simulink model "ards_model"  (R2020b)
settings: Solver=VariableStepAuto  StartTime=0.0  StopTime=480  MaxStep=0.2  RelTol=1e-3
model workspace: external: MAT-File model_workspace.mat (data not in the file)
values from neighbouring files (symbols this model uses):
  C_a_CO2_0 = 0.54    [model_workspace.mat]
  C_a_O2_0 = 0.1974    [model_workspace.mat]
  C_v_CO2_0 = 0.72    [model_workspace.mat]
  C_v_O2_0 = 0.13    [model_workspace.mat]
  moving_average_period = 5    [model_workspace.mat]
  P_ap_0 = 15    [model_workspace.mat]
  P_as_0 = 105.55    [model_workspace.mat]
  P_default = [105.55 4 15 6]    [model_workspace.mat]
  P_vs_0 = 4    [model_workspace.mat]
  Q_0 = 4.8    [model_workspace.mat]
undefined symbols (not defined in the file or in its folder): cRS, Pinsp, VT
libraries: pid_lib x1
(part 1 of 3)
settings Model: OrderedModelArguments=off  Creator=RH  LastModifiedBy=fonck
settings DebuggingCC: SignalInfNanChecking=warning  AlgebraicLoopMsg=none  ArtificialAlgebraicLoopMsg=none  UnconnectedInputMsg=none  UnconnectedOutputMsg=none  UnconnectedLineMsg=none  UniqueDataStoreMsg=error  BusObjectLabelMismatch=none

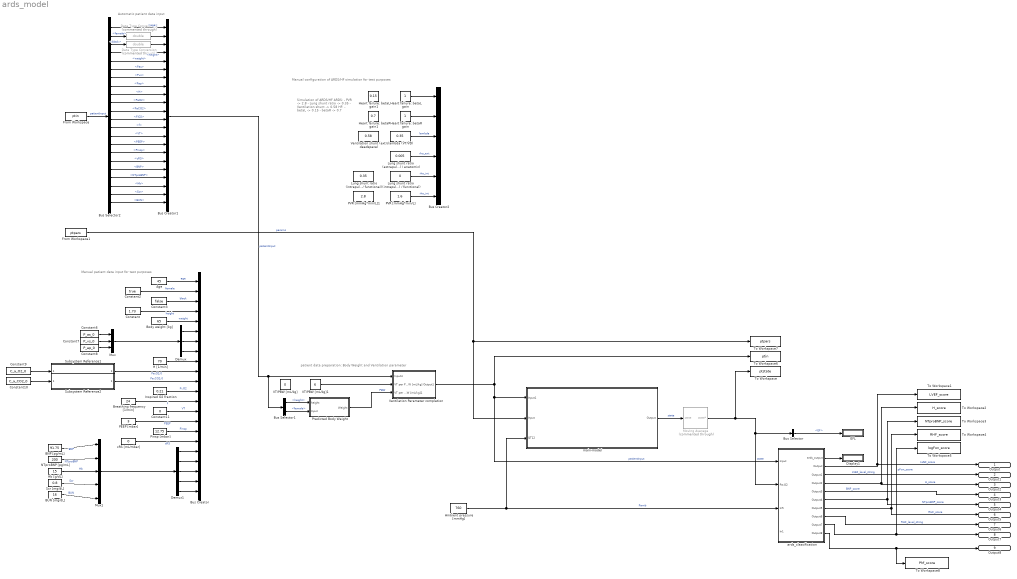
== system ards_model ==
  note: patient data preparation: Body Weight and Ventilation parameter
  note: Manual configuration of ARDS/HF simulation for test purposes
  note: Automatic patient data input
  note: Manual patient data input for test purposes
  note: Simulation of ARDS/HF
      | ARDS:
      | - PVR -> 2.8
      | - Lung shunt ratio -> 0.35
      | - Ventilation shunt -> 0.58
      | HF:
      | - betaL -> 0.15
      | - betaR -> 0.7
  Age : Constant  Value=45
  Ambient pressure [mmHg] : Constant  Value=760
  BNP [pg/mL] : Constant  Value=91.75
  BUN [mg/dL] : Constant  Value=16
  Body weight [kg] : Constant  Value=65  OutDataTypeStr=double
  Breathing frequency [1/min] : Constant  Value=24
  Bus Creator : BusCreator  Inputs=22  OutDataTypeStr=Bus: PatientInput
      settings: InheritFromInputs=off
  Bus Creator1 : BusCreator  Inputs=22  OutDataTypeStr=Bus: PatientInput
      settings: InheritFromInputs=off
  Bus Creator2 : BusCreator  Inputs=6  OutDataTypeStr=Bus: PatientParams
      settings: InheritFromInputs=off
  Bus Selector : BusSelector  OutputSignals=cvs.LV.EF
  Bus Selector1 : BusSelector  OutputSignals=height,female
  Bus Selector2 : BusSelector  OutputSignals=age,female,black,height,weight,Pas,Pvs,Pap,H,PaO2,PaCO2,FiO2,f,VT,PEEP,Pinsp,cRS,BNP,NTproBNP,Hb,Scr,BUN
  Constant : Constant  Value=1.73
  Constant10 : Constant  Value=C_a_CO2_0
  Constant11 : Constant  Value=0
  Constant2 : Constant  Value=true
  Constant3 : Constant  Value=false
  Constant6 : Constant  Value=P_as_0
  Constant7 : Constant  Value=P_vs_0
  Constant8 : Constant  Value=P_ap_0
  Constant9 : Constant  Value=C_a_O2_0
  Data Type Conversion : DataTypeConversion  Commented=through  OutDataTypeStr=double
  Data Type Conversion1 : DataTypeConversion  Commented=through  OutDataTypeStr=double
  Demux : Demux  Outputs=3
  Demux1 : Demux  Outputs=5
  Display1 : Display
  EFL : Display
  From Workspace : FromWorkspace  VariableName=ptin  OutDataTypeStr=Bus: PatientInput  OutputAfterFinalValue=Holding final value
  From Workspace1 : FromWorkspace  VariableName=ptpars  OutDataTypeStr=Bus: PatientParams  OutputAfterFinalValue=Holding final value
  H [1/min] : Constant  Value=70
  Hb [g/dL] : Constant  Value=15
  Heart failure: betaL gain : Constant
  Heart failure: betaL gain1 : Constant  Value=0.15
  Heart failure: betaR gain : Constant
  Heart failure: betaR gain1 : Constant  Value=0.7
  Inspired O2 fraction : Constant  Value=0.21
  Lung shunt ratio (extrapulmonal / anatomic) : Constant  Value=0.005
  Lung shunt ratio (intrapulmonal / functional) : Constant  Value=0
  Lung shunt ratio (intrapulmonal / functional)1 : Constant  Value=0.35
  Moving Average : Subsystem  Commented=through
  Mux : Mux  Inputs=3
  Mux1 : Mux  Inputs=5
  NTproBNP [pg/mL] : Constant  Value=200
  PEEP [mbar] : Constant  Value=3
  PVR [mmHg*min/L] : Constant  Value=1.6
  PVR [mmHg*min/L]1 : Constant  Value=2.8
  Pinsp [mbar] : Constant  Value=12.75
  Predicted Body Weight : Subsystem  TreatAsAtomicUnit=on
  Scr [mg/dL] : Constant  Value=0.8
  Subsystem Reference1 : Subsystem  ReferencedSubsystem=O2_dissociation_inv
  Subsystem Reference2 : Subsystem  ReferencedSubsystem=CO2_dissociation_inv
  To Workspace : ToWorkspace  VariableName=ptstate  SaveFormat=Timeseries  SampleTime=-1
  To Workspace1 : ToWorkspace  VariableName=LVEF_score  SaveFormat=Timeseries  SampleTime=-1
  To Workspace2 : ToWorkspace  VariableName=H_score  SaveFormat=Timeseries  SampleTime=-1
  To Workspace3 : ToWorkspace  VariableName=NTproBNP_score  SaveFormat=Timeseries  SampleTime=-1
  To Workspace4 : ToWorkspace  VariableName=RHF_score  SaveFormat=Timeseries  SampleTime=-1
  To Workspace5 : ToWorkspace  VariableName=logFon_score  SaveFormat=Timeseries  SampleTime=-1
  To Workspace6 : ToWorkspace  VariableName=ptin  SaveFormat=Timeseries  SampleTime=-1
  To Workspace7 : ToWorkspace  VariableName=ptpars  SaveFormat=Timeseries  SampleTime=-1
  To Workspace8 : ToWorkspace  VariableName=Phf_score  SaveFormat=Timeseries  SampleTime=-1
  VT/PBW [mL/kg] : Constant  Value=0
  VT/PBW [mL/kg]1 : Constant  Value=6
  Ventilation Parameter completion : Subsystem
  Ventilation shunt (extra deadspace) : Constant  Value=0.58
  ards_classification : Subsystem
  cRS [mL/mbar] : Constant  Value=0
  lambda (VT/VD) : Constant  Value=0.35
  main-model : Subsystem
  Output : Outport
  Output1 : Outport  Port=2
  Output2 : Outport  Port=3
  Output3 : Outport  Port=4
  Output4 : Outport  Port=5
  Output5 : Outport  Port=6
  Output6 : Outport  Port=7
  Output7 : Outport  Port=8
  Output8 : Outport  Port=9
  wires:
  Breathing frequency [1/min]/1 -> Bus Creator/13  "f"
  Ambient pressure [mmHg]/1 -> main-model/3(QT12), ards_classification/3(In5)  "Pamb"
  Inspired O2 fraction/1 -> Bus Creator/12  "Fi;O2"
  Constant2/1 -> Bus Creator/2  "female"
  Constant3/1 -> Bus Creator/3  "black"
  H [1/min]/1 -> Bus Creator/9
  Bus Selector1/1 -> Predicted Body Weight/1(height)  "<height>"
  Predicted Body Weight/1(Weight) -> Ventilation Parameter completion/3(VT per PBW [mL/kg]1)  "PBW"
  Bus Selector1/2 -> Predicted Body Weight/2(Input)  "<female>"
  VT/PBW [mL/kg]1/1 -> Ventilation Parameter completion/2(VT per PBW [mL/kg])
  Bus Creator1/1 -> Bus Selector1/1, Ventilation Parameter completion/1(Input4)  "patientInput"
  Body weight [kg]/1 -> Bus Creator/5  "weight"
  Age/1 -> Bus Creator/1  "age"
  Demux/1 -> Bus Creator/6
  Demux/2 -> Bus Creator/7
  Demux/3 -> Bus Creator/8
  Constant6/1 -> Mux/1
  Constant7/1 -> Mux/2
  Constant8/1 -> Mux/3
  Mux/1 -> Demux/1
  Subsystem Reference1/1 -> Bus Creator/10  "Pa;O2;0"
  Subsystem Reference2/1 -> Bus Creator/11  "Pa;CO2;0"
  Constant9/1 -> Subsystem Reference1/1
  Constant10/1 -> Subsystem Reference2/1
  Constant11/1 -> Bus Creator/14  "VT"
  PEEP [mbar]/1 -> Bus Creator/15  "PEEP"
  Pinsp [mbar]/1 -> Bus Creator/16  "Pinsp"
  cRS [mL/mbar]/1 -> Bus Creator/17  "cRS"
  Ventilation Parameter completion/1(Output1) -> To Workspace6/1, main-model/1(Input1), ards_classification/1(Input)  "patientInput"
  Scr [mg/dL]/1 -> Mux1/4  "Scr"
  NTproBNP [pg/mL]/1 -> Mux1/2  "NTproBNP"
  Hb [g/dL]/1 -> Mux1/3  "Hb"
  BNP [pg/mL]/1 -> Mux1/1  "BNP"
  Demux1/4 -> Bus Creator/21
  Demux1/1 -> Bus Creator/18
  Demux1/2 -> Bus Creator/19
  Demux1/3 -> Bus Creator/20
  Mux1/1 -> Demux1/1
  Bus Selector/1 -> EFL/1  "<EF>"
  Constant/1 -> Bus Creator/4  "height"
  main-model/1(Output) -> Moving Average/1(state)  "state"
  Moving Average/1(state*) -> To Workspace/1, Bus Selector/1, ards_classification/2(Pa;O2)  "state"
  Heart failure: betaR gain/1 -> Bus Creator2/2
  Heart failure: betaL gain/1 -> Bus Creator2/1
  lambda (VT/VD)/1 -> Bus Creator2/3  "lambda"
  Lung shunt ratio (extrapulmonal / anatomic)/1 -> Bus Creator2/4  "rho_ext"
  Lung shunt ratio (intrapulmonal / functional)/1 -> Bus Creator2/5  "rho_int"
  From Workspace1/1 -> To Workspace7/1, main-model/2(Input)  "params"
  PVR [mmHg*min/L]/1 -> Bus Creator2/6  "rho_int"
  BUN [mg/dL]/1 -> Mux1/5  "BUN"
  Demux1/5 -> Bus Creator/22
  ards_classification/2(Output) -> Output/1, To Workspace1/1  "LVEF_score"
  ards_classification/3(Output1) -> Output1/1  "LVEF_level_string"
  ards_classification/9(Output7) -> To Workspace5/1, Output7/1  "pFon_score"
  ards_classification/8(Output6) -> Output6/1  "RHF_level_string"
  ards_classification/7(Output5) -> Output5/1, To Workspace4/1  "RHF_score"
  ards_classification/6(Output4) -> Output4/1, To Workspace3/1  "NTproBNP_score"
  ards_classification/5(Output3) -> Output3/1  "BNP_score"
  ards_classification/4(Output2) -> Output2/1, To Workspace2/1  "H_score"
  Bus Selector2/21 -> Bus Creator1/21  "<Scr>"
  Bus Selector2/22 -> Bus Creator1/22  "<BUN>"
  Bus Selector2/19 -> Bus Creator1/19  "<NTproBNP>"
  Bus Selector2/20 -> Bus Creator1/20  "<Hb>"
  Bus Selector2/18 -> Bus Creator1/18  "<BNP>"
  Bus Selector2/16 -> Bus Creator1/16  "<Pinsp>"
  Bus Selector2/17 -> Bus Creator1/17  "<cRS>"
  Bus Selector2/15 -> Bus Creator1/15  "<PEEP>"
  Bus Selector2/14 -> Bus Creator1/14  "<VT>"
  Bus Selector2/12 -> Bus Creator1/12  "<FiO2>"
  Bus Selector2/11 -> Bus Creator1/11  "<PaCO2>"
  Bus Selector2/13 -> Bus Creator1/13  "<f>"
  Bus Selector2/9 -> Bus Creator1/9  "<H>"
  Bus Selector2/8 -> Bus Creator1/8  "<Pap>"
  Bus Selector2/10 -> Bus Creator1/10  "<PaO2>"
  Bus Selector2/7 -> Bus Creator1/7  "<Pvs>"
  Bus Selector2/6 -> Bus Creator1/6  "<Pas>"
  Bus Selector2/4 -> Bus Creator1/4  "<height>"
  Bus Selector2/5 -> Bus Creator1/5  "<weight>"
  Bus Selector2/1 -> Bus Creator1/1  "<age>"
  Bus Selector2/2 -> Data Type Conversion1/1  "<female>"
  Bus Selector2/3 -> Data Type Conversion/1  "<black>"
  Data Type Conversion/1 -> Bus Creator1/3
  Data Type Conversion1/1 -> Bus Creator1/2
  From Workspace/1 -> Bus Selector2/1  "patientInput"
  ards_classification/1(ards_output) -> Display1/1
  ards_classification/10(Output8) -> To Workspace8/1, Output8/1

== system ards_model/Moving Average ==
  state : Inport
  Bus to Vector : BusToVector
  Gain : Gain  Gain=1/moving_average_period
  Integrator : Integrator
  Subsystem : Subsystem  ReferencedSubsystem=patient_state_to_bus
  Subtract : Sum  Inputs=+-
  Transport Delay : TransportDelay  DelayTime=moving_average_period
  state* : Outport  OutDataTypeStr=Bus: PatientState
  wires:
  Integrator/1 -> Subtract/1, Transport Delay/1
  state/1 -> Bus to Vector/1
  Subtract/1 -> Gain/1
  Transport Delay/1 -> Subtract/2
  Bus to Vector/1 -> Integrator/1
  Gain/1 -> Subsystem/1
  Subsystem/1 -> state*/1

== system ards_model/Predicted Body Weight ==
  note: Predicted body weight
      | Source: Ventilation with lower tidal volumes [...], page 3
  height : Inport  Unit=m
  Input : Inport  Port=2  OutDataTypeStr=boolean
  Add4 : Sum  Inputs=+-
  Constant1 : Constant  Value=1.524
  Constant3 : Constant  Value=0
  Gain : Gain  Gain=91
  IfThenElse : Subsystem
  Max : MinMax  Function=max  Inputs=2
  Subtract1 : Sum
  female : Constant  Value=45.5
  male : Constant  Value=50
  Weight : Outport  Unit=kg
  wires:
  Max/1 -> Gain/1
  Constant1/1 -> Add4/2
  Gain/1 -> Subtract1/1
  Constant3/1 -> Max/2
  height/1 -> Add4/1  "height"
  Subtract1/1 -> Weight/1  "PBW"
  Add4/1 -> Max/1
  female/1 -> IfThenElse/2(then)
  male/1 -> IfThenElse/3(else)
  IfThenElse/1(out) -> Subtract1/2
  Input/1 -> IfThenElse/1(if)  "female"

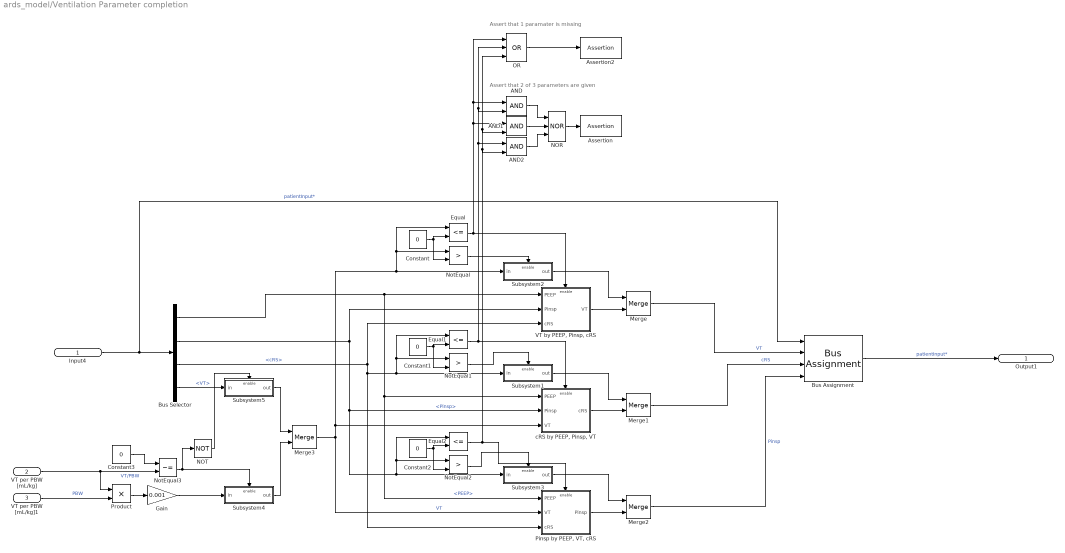
== system ards_model/Ventilation Parameter completion ==
  note: Assert that 2 of 3 parameters are given
  note: Assert that 1 paramater is missing
  Input4 : Inport  OutDataTypeStr=Bus: PatientInput
  VT per PBW [mL/kg] : Inport  Port=2  Unit=mL/kg
  VT per PBW [mL/kg]1 : Inport  Port=3  Unit=kg
  AND : Logic  IconShape=distinctive  AllPortsSameDT=off  OutDataTypeStr=boolean
  AND1 : Logic  IconShape=distinctive  AllPortsSameDT=off  OutDataTypeStr=boolean
  AND2 : Logic  IconShape=distinctive  AllPortsSameDT=off  OutDataTypeStr=boolean
  Assertion : Assertion
  Assertion2 : Assertion
  Bus Assignment : BusAssignment  AssignedSignals=VT,cRS,Pinsp
  Bus Selector : BusSelector  OutputSignals=PEEP,Pinsp,cRS,VT
  Constant{,1..3} (4 alike) : Constant  Value=0
  Equal : RelationalOperator  Operator=<=  OutDataTypeStr=boolean  RndMeth=Simplest
  Equal1 : RelationalOperator  Operator=<=  OutDataTypeStr=boolean  RndMeth=Simplest
  Equal2 : RelationalOperator  Operator=<=  OutDataTypeStr=boolean  RndMeth=Simplest
  Gain : Gain  Gain=0.001
  Merge{,1..3} (4 alike) : Merge
  NOR : Logic  Operator=NOR  Inputs=3  IconShape=distinctive  AllPortsSameDT=off  OutDataTypeStr=boolean
  NOT : Logic  Operator=NOT  IconShape=distinctive  AllPortsSameDT=off  OutDataTypeStr=boolean
  NotEqual : RelationalOperator  Operator=>  OutDataTypeStr=boolean  RndMeth=Simplest
  NotEqual1 : RelationalOperator  Operator=>  OutDataTypeStr=boolean  RndMeth=Simplest
  NotEqual2 : RelationalOperator  Operator=>  OutDataTypeStr=boolean  RndMeth=Simplest
  NotEqual3 : RelationalOperator  Operator=~=  OutDataTypeStr=boolean  RndMeth=Simplest
  OR : Logic  Operator=OR  Inputs=3  IconShape=distinctive  AllPortsSameDT=off  OutDataTypeStr=boolean
  "Pinsp by PEEP, VT, cRS" : Subsystem
  Product : Product
  Subsystem1 : Subsystem
  Subsystem2 : Subsystem
  Subsystem3 : Subsystem
  Subsystem4 : Subsystem
  Subsystem5 : Subsystem
  "VT by PEEP, Pinsp, cRS" : Subsystem
  "cRS by PEEP, Pinsp, VT" : Subsystem
  Output1 : Outport  OutDataTypeStr=Bus: PatientInput
  wires:
  Equal/1 -> OR/1, AND/1, AND1/1, "VT by PEEP, Pinsp, cRS"/Enable
  "VT by PEEP, Pinsp, cRS"/1(VT) -> Merge/2
  Bus Selector/1 -> "cRS by PEEP, Pinsp, VT"/1(PEEP), "Pinsp by PEEP, VT, cRS"/1(PEEP), "VT by PEEP, Pinsp, cRS"/1(PEEP)  "<PEEP>"
  NotEqual2/1 -> Subsystem3/Enable
  Merge3/1 -> Subsystem2/1(in), NotEqual/1, Equal/1, "cRS by PEEP, Pinsp, VT"/3(VT), "Pinsp by PEEP, VT, cRS"/2(VT)  "VT"
  Subsystem2/1(out) -> Merge/1
  Merge2/1 -> Bus Assignment/4  "Pinsp"
  Subsystem1/1(out) -> Merge1/1
  "cRS by PEEP, Pinsp, VT"/1(cRS) -> Merge1/2
  NotEqual1/1 -> Subsystem1/Enable
  "Pinsp by PEEP, VT, cRS"/1(Pinsp) -> Merge2/2
  Equal2/1 -> OR/3, AND1/2, AND2/2, "Pinsp by PEEP, VT, cRS"/Enable
  Equal1/1 -> AND2/1, OR/2, AND/2, "cRS by PEEP, Pinsp, VT"/Enable
  Merge1/1 -> Bus Assignment/3  "cRS"
  Subsystem3/1(out) -> Merge2/1
  Merge/1 -> Bus Assignment/2  "VT"
  NotEqual/1 -> Subsystem2/Enable
  AND1/1 -> NOR/2
  AND/1 -> NOR/1
  AND2/1 -> NOR/3
  NOR/1 -> Assertion/1
  OR/1 -> Assertion2/1
  Constant/1 -> Equal/2, NotEqual/2
  VT per PBW [mL/kg]/1 -> NotEqual3/2, Product/1  "VT/PBW"
  VT per PBW [mL/kg]1/1 -> Product/2  "PBW"
  Constant3/1 -> NotEqual3/1
  NotEqual3/1 -> Subsystem4/Enable, NOT/1
  Product/1 -> Gain/1
  Gain/1 -> Subsystem4/1(in)
  Subsystem5/1(out) -> Merge3/1
  Subsystem4/1(out) -> Merge3/2
  NOT/1 -> Subsystem5/Enable
  Bus Selector/4 -> Subsystem5/1(in)  "<VT>"
  Input4/1 -> Bus Assignment/1, Bus Selector/1  "patientInput*"
  Constant1/1 -> Equal1/2, NotEqual1/2
  Bus Selector/3 -> "VT by PEEP, Pinsp, cRS"/3(cRS), "Pinsp by PEEP, VT, cRS"/3(cRS), Subsystem1/1(in), NotEqual1/1, Equal1/1  "<cRS>"
  Bus Selector/2 -> "VT by PEEP, Pinsp, cRS"/2(Pinsp), Subsystem3/1(in), Equal2/1, NotEqual2/1, "cRS by PEEP, Pinsp, VT"/2(Pinsp)  "<Pinsp>"
  Constant2/1 -> NotEqual2/2, Equal2/2
  Bus Assignment/1 -> Output1/1  "patientInput*"

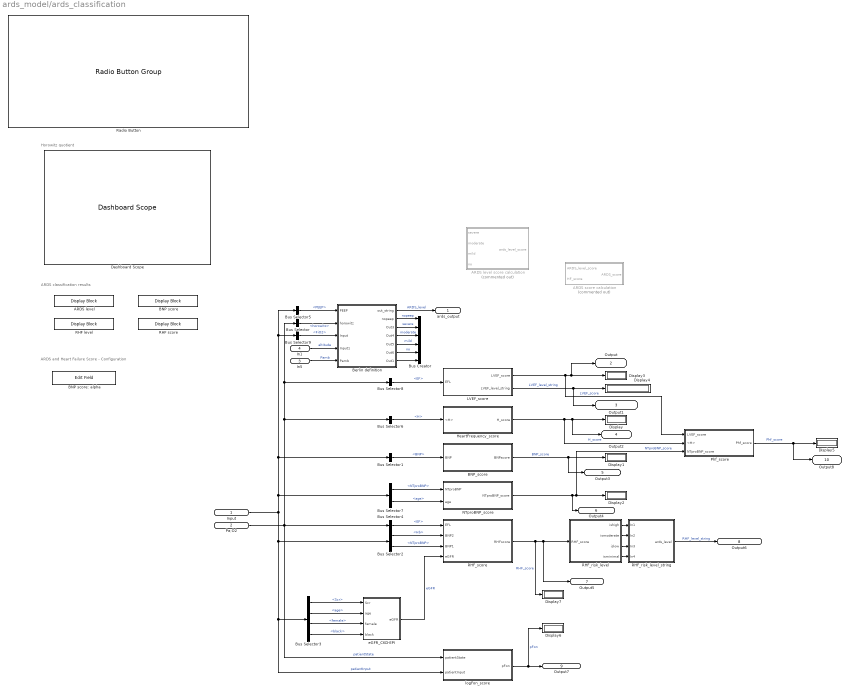
== system ards_model/ards_classification ==
  note: ARDS classification results
  note: ARDS and Heart Failure Score - Configuration
  note: Horowitz quotient
  Input : Inport  OutDataTypeStr=Bus: PatientInput
  Pa;O2 : Inport  Port=2  OutDataTypeStr=Bus: PatientState
  In5 : Inport  Port=3  Unit=mmHg
  In1 : Inport  Port=4  Unit=m
  ARDS level : DisplayBlock  LabelPosition=Hide  Format=short  Transparency=1
  ARDS level score calculation : Subsystem  Commented=on
  ARDS score calculation : Subsystem  Commented=on
  BNP score : DisplayBlock  LabelPosition=Hide  Format=short  Transparency=1
  BNP score: alpha : EditField  LabelPosition=Hide  ShowInitialText=on  Alignment=Center
  BNP_score : Subsystem
  Berlin definition : Subsystem
  Bus Creator : BusCreator  Inputs=6
  Bus Selector : BusSelector  OutputSignals=rs.horowitz
  Bus Selector1 : BusSelector  OutputSignals=BNP
  Bus Selector2 : BusSelector  OutputSignals=Hb,NTproBNP
  Bus Selector3 : BusSelector  OutputSignals=Scr,age,female,black
  Bus Selector4 : BusSelector  OutputSignals=cvs.LV.EF
  Bus Selector5 : BusSelector  OutputSignals=PEEP
  Bus Selector6 : BusSelector  OutputSignals=cvs.H
  Bus Selector7 : BusSelector  OutputSignals=NTproBNP,age
  Bus Selector8 : BusSelector  OutputSignals=cvs.LV.EF
  Bus Selector9 : BusSelector  OutputSignals=FiO2
  Dashboard Scope : DashboardScope  ShowInitialText=off  Ymin=0  Ymax=750
  Display{,1..7} (8 alike) : Display
  HeartFrequency_score : Subsystem
  LVEF_score : Subsystem
  NTproBNP_score : Subsystem
  Phf_score : Subsystem
  RHF level : DisplayBlock  LabelPosition=Hide  Format=short  Transparency=1
  RHF score : DisplayBlock  LabelPosition=Hide  Format=short  Transparency=1
  RHF_risk_level : Subsystem
  RHF_risk_level_string : Subsystem
  RHF_score : Subsystem
  Radio Button : RadioButtonGroup  LabelPosition=Hide  SelectedLabel=Pérez-Padilla et al. (altitude)  ButtonGroupName=Horowitz correction mode
      settings: Values={{'Pérez-Padilla et al. (altitude)', 'Pérez-Padilla et al. (Pamb)', 'Berlin Definition (original)', 'Berlin Definition (reciprocal)'}, [1 2 3 4]}
  eGFR_CKD-EPI : Subsystem
  logFon_score : Subsystem
  ards_output : Outport
  Output : Outport  Port=2
  Output1 : Outport  Port=3
  Output2 : Outport  Port=4
  Output3 : Outport  Port=5
  Output4 : Outport  Port=6
  Output5 : Outport  Port=7
  Output6 : Outport  Port=8
  Output7 : Outport  Port=9
  Output8 : Outport  Port=10
  wires:
  Bus Selector1/1 -> BNP_score/1(BNP)  "<BNP>"
  Berlin definition/1(out_string) -> ards_output/1  "ARDS_level"
  Pa;O2/1 -> logFon_score/1(patientState), Bus Selector8/1, Bus Selector/1, Bus Selector6/1, Bus Selector4/1  "patientState"
  In5/1 -> Berlin definition/5(Pamb)  "Pamb"
  Bus Selector/1 -> Berlin definition/2(horowitz)  "<horowitz>"
  RHF_risk_level/1(ishigh) -> RHF_risk_level_string/1(In1)
  RHF_risk_level/2(ismoderate) -> RHF_risk_level_string/2(In2)
  RHF_risk_level/3(islow) -> RHF_risk_level_string/3(In3)
  RHF_risk_level/4(isminimal) -> RHF_risk_level_string/4(In4)
  Bus Selector2/1 -> RHF_score/2(BNP2)  "<Hb>"
  Bus Selector2/2 -> RHF_score/3(BNP1)  "<NTproBNP>"
  eGFR_CKD-EPI/1(eGFR) -> RHF_score/4(eGFR)  "eGFR"
  RHF_score/1(RHFscore) -> Display7/1, Output5/1, RHF_risk_level/1(RHF_score)  "RHF_score"
  Input/1 -> Bus Selector1/1, Bus Selector9/1, Bus Selector5/1, Bus Selector7/1, Bus Selector2/1, logFon_score/2(patientInput), Bus Selector3/1  "patientInput"
  Bus Selector3/1 -> eGFR_CKD-EPI/1(Scr)  "<Scr>"
  Bus Selector3/2 -> eGFR_CKD-EPI/2(age)  "<age>"
  Bus Selector3/4 -> eGFR_CKD-EPI/4(black)  "<black>"
  Bus Selector3/3 -> eGFR_CKD-EPI/3(female)  "<female>"
  Berlin definition/2(nopeep) -> Bus Creator/1  "nopeep"
  Berlin definition/3(Out3) -> Bus Creator/2  "severe"
  Berlin definition/4(Out4) -> Bus Creator/3  "moderate"
  Berlin definition/5(Out5) -> Bus Creator/4  "mild"
  Berlin definition/6(Out6) -> Bus Creator/5  "no"
  Berlin definition/7(Out1) -> Bus Creator/6
  Bus Selector4/1 -> RHF_score/1(EFL)  "<EF>"
  Bus Selector5/1 -> Berlin definition/1(PEEP)  "<PEEP>"
  Bus Selector6/1 -> HeartFrequency_score/1(<H>)  "<H>"
  Bus Selector7/1 -> NTproBNP_score/1(NTproBNP)  "<NTproBNP>"
  Bus Selector7/2 -> NTproBNP_score/2(age)  "<age>"
  HeartFrequency_score/1(H_score) -> Phf_score/2(<H>), Output2/1, Display/1  "H_score"
  BNP_score/1(BNPscore) -> Output3/1, Display1/1  "BNP_score"
  NTproBNP_score/1(NTproBNP_score) -> Phf_score/3(NTproBNP_score), Display2/1, Output4/1  "NTproBNP_score"
  LVEF_score/1(LVEF_score) -> Display3/1, Output/1, Phf_score/1(LVEF_score)  "LVEF_score"
  LVEF_score/2(LVEF_level_string) -> Output1/1, Display4/1  "LVEF_level_string"
  Bus Selector8/1 -> LVEF_score/1(EFL)  "<EF>"
  RHF_risk_level_string/1(ards_level) -> Output6/1  "RHF_level_string"
  logFon_score/1(pFon) -> Display6/1, Output7/1  "pFon"
  Bus Selector9/1 -> Berlin definition/3(Input)  "<FiO2>"
  In1/1 -> Berlin definition/4(Input1)  "altitude"
  Phf_score/1(Phf_score) -> Output8/1, Display5/1  "Phf_score"

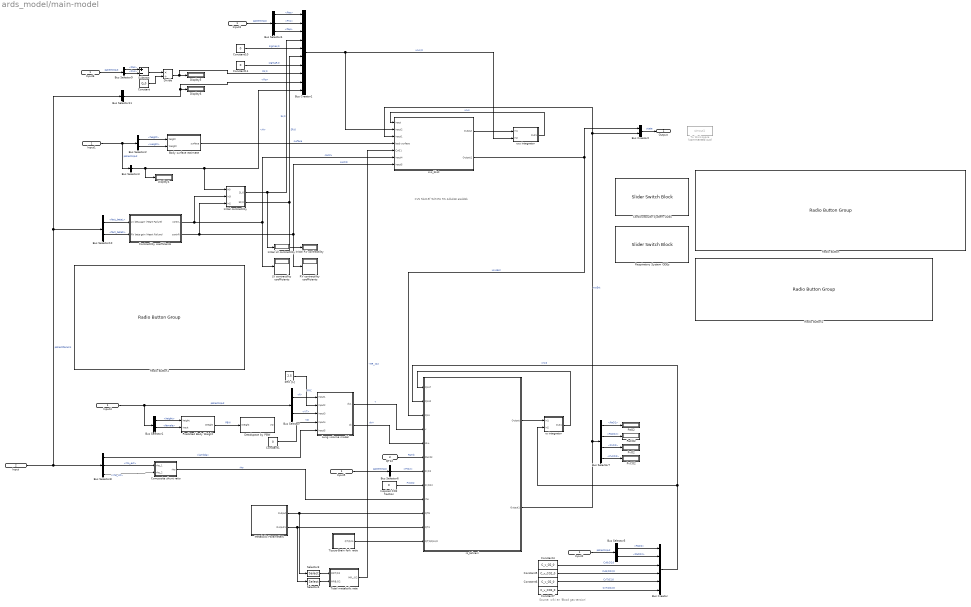
== system ards_model/main-model ==
  note: Source: wiki en 'Blood gas tension'
  note: CVS 5b215f 9d729c
      | RS 4dbd38 a6dd8b
  Input1 : Inport  OutDataTypeStr=Bus: PatientInput
  Input : Inport  Port=2  OutDataTypeStr=Bus: PatientParams  PortDimensions=6
  QT12 : Inport  Port=3  Unit=mmHg
  Body surface estimate : Subsystem  TreatAsAtomicUnit=on
  Bus Creator : BusCreator  Inputs=6  OutDataTypeStr=Bus: RespiratoryState
      settings: InheritFromInputs=off
  Bus Creator1 : BusCreator  Inputs=10  OutDataTypeStr=Bus: CardioVascularState
      settings: InheritFromInputs=off
  Bus Creator2 : BusCreator  Inputs=2  OutDataTypeStr=Bus: PatientState
      settings: InheritFromInputs=off
  Bus Selector : BusSelector  OutputSignals=f,VT
  Bus Selector1 : BusSelector  OutputSignals=height,female
  Bus Selector10 : BusSelector  OutputSignals=fact_betaL,fact_betaR
  Bus Selector11 : BusSelector  OutputSignals=Rp
  Bus Selector2 : BusSelector  OutputSignals=height,weight
  Bus Selector3 : BusSelector  OutputSignals=H
  Bus Selector4 : BusSelector  OutputSignals=Pas,Pvs,Pap
  Bus Selector5 : BusSelector  OutputSignals=PaO2,PaCO2
  Bus Selector6 : BusSelector  OutputSignals=FiO2
  Bus Selector7 : BusSelector  OutputSignals=PaO2,PaCO2,PvO2,PvCO2
  Bus Selector8 : BusSelector  OutputSignals=lambda,rho_ext,rho_int
  Bus Selector9 : BusSelector  OutputSignals=Pas,Pvs
  Cardiovascular System ODEs : SliderSwitchBlock
      settings: Values={{'Off', 'On'}, [0 1]}
  Composite shunt ratio : Subsystem
  Constant : Constant  Value=Q_0
  Constant1 : Constant  Value=0
  Constant10 : Constant  Value=0
  Constant11 : Constant  Value=0
  Constant4 : Constant  Value=C_v_O2_0
  Constant5 : Constant  Value=C_v_CO2_0
  Constant6 : Constant  Value=C_v_O2_0
  Constant7 : Constant  Value=C_v_CO2_0
  Contractility coefficients : Subsystem
  Deadspace by PBW : Subsystem  TreatAsAtomicUnit=on
  Display4 : Display
  Display5 : Display
  Display6 : Display
  Divide : Product  Inputs=*/
  FRC [L] : Constant  Value=2.5
  Initial LV contractility : Display
  Initial RV contractility : Display
  Initial contractility : Subsystem
  Input{2..6} (5 alike) : InportShadow  OutDataTypeStr=Bus: PatientInput
  Inspired CO2 fraction : Constant  Value=0
  LV contractility coefficients : Display
  Lung volume model : Subsystem  TreatAsAtomicUnit=on
  Metabolic Parameters : Subsystem
  PaCO2 : Display
  PaO2 : Display
  Predicted Body Weight : Subsystem  TreatAsAtomicUnit=on
  PvCO2 : Display
  PvO2 : Display
  RV contractility coefficients : Display
  Radio Button : RadioButtonGroup  LabelPosition=Hide  SelectedLabel=ODE from [BKST (1.27)]: By Metabolic rates and Ca;O2  ButtonGroupName=Systemic vascular resistance: Calculation mode
      settings: Values={{'Constant', 'Linear relation from [BKST (1.24)]: By Cv;O2', 'ODE from [BKST (1.27)]: By Metabolic rates and Ca;O2'}, [0 1 2]}
  Radio Button1 : RadioButtonGroup  LabelPosition=Hide  SelectedLabel=from table 3.1 (healthy)  ButtonGroupName=Contractility coefficient selection (see [BKST] table 1.5)
      settings: Values={{'without QL measurements', 'with QL measurements', 'with QL measurements, "exact" gradients', 'from table 3.1 (healthy)', 'from table 3.1 (Heart Failure)'}, [1 2 3 4 5]}
  Radio Button2 : RadioButtonGroup  LabelPosition=Hide  SelectedLabel=Linear relationship with Heart Frequency (H)  ButtonGroupName=Heart Contractility: Calculation mode
      settings: Values={{'Linear relationship with Heart Frequency (H)', 'Second-order ODE'}, [0 1]}
  Respiratory System ODEs : SliderSwitchBlock
      settings: Values={{'Off', 'On'}, [0 1]}
  Selector3 : Selector  InputPortWidth=3  IndexOptions=Index vector (dialog)  Indices=2  OutputSizes=1
  Selector4 : Selector  InputPortWidth=3  IndexOptions=Index vector (dialog)  Indices=2  OutputSizes=1
  Subtract : Sum  Inputs=+-
  Tissue-Brain fork ratio : Subsystem
  To Workspace : ToWorkspace  Commented=on  VariableName=simout1  SaveFormat=Timeseries  SampleTime=-1
      settings: MaxDataPoints=1
  Total metabolic rate : Subsystem
  cvs integrator : Subsystem
  cvs_bkst : Subsystem
  rs integrator : Subsystem
  rs_tehrani : Subsystem  TreatAsAtomicUnit=on
  Output : Outport  OutDataTypeStr=Bus: PatientState
  wires:
  Divide/1 -> Bus Creator1/8, Display5/1  "Rs;0"
  Bus Selector9/2 -> Subtract/2  "<Pvs>"
  Bus Selector9/1 -> Subtract/1  "<Pas>"
  Input5/1 -> Bus Selector6/1  "patientInput"
  Input2/1 -> Bus Selector5/1  "patientInput"
  Bus Selector/2 -> Lung volume model/3(Input3)  "<VT>"
  Bus Selector7/1 -> PaO2/1  "<PaO2>"
  Bus Selector7/3 -> PvO2/1  "<PvO2>"
  Input1/1 -> Bus Selector2/1, Bus Selector3/1  "patientInput"
  Bus Selector7/2 -> PaCO2/1  "<PaCO2>"
  Bus Selector5/2 -> Bus Creator/2  "<PaCO2>"
  cvs_bkst/2(Output1) -> Bus Creator2/1, rs_tehrani/3(Qco)  "xcvsExt"
  Bus Creator2/1 -> Output/1  "state"
  Contractility coefficients/1(contrL) -> cvs_bkst/6(Input4), LV contractility coefficients/1, Initial contractility/2(In3)  "contrL"
  cvs integrator/1(Out1) -> cvs_bkst/1(Input)  "xcvs"
  Contractility coefficients/2(contrR) -> cvs_bkst/7(Input5), RV contractility coefficients/1, Initial contractility/3(In2)  "contrR"
  cvs_bkst/1(Output) -> cvs integrator/1(In1)
  rs_tehrani/2(Output1) -> Bus Creator2/2, cvs_bkst/3(Input1), Bus Selector7/1  "xrsExt"
  Bus Selector4/3 -> Bus Creator1/3  "<Pap>"
  Bus Selector4/1 -> Bus Creator1/1  "<Pas>"
  Bus Selector11/1 -> Bus Creator1/9, Display6/1  "<Rp>"
  Bus Creator1/1 -> cvs integrator/2(In2), cvs_bkst/2(Input2)  "xcvs;0"
  Total metabolic rate/1(MR_;O2) -> cvs_bkst/5(CvO1)  "-MR_;O2"
  Bus Selector7/4 -> PvCO2/1  "<PvCO2>"
  Constant10/1 -> Bus Creator1/5  "sigmaL;0"
  Bus Selector10/1 -> Contractility coefficients/1(LV beta gain (Heart Failure))  "<fact_betaL>"
  Bus Selector1/2 -> Predicted Body Weight/2(Input)  "<female>"
  Constant11/1 -> Bus Creator1/7  "sigmaR;0"
  Bus Selector4/2 -> Bus Creator1/2  "<Pvs>"
  Initial contractility/1(SL;0) -> Initial LV contractility/1, Bus Creator1/4  "SL;0"
  Bus Selector10/2 -> Contractility coefficients/2(RV beta gain (Heart Failure))  "<fact_betaR>"
  Input3/1 -> Bus Selector4/1  "patientInput"
  Input6/1 -> Bus Selector9/1  "patientInput"
  rs integrator/1(Out1) -> rs_tehrani/1(Qco7)
  Bus Selector5/1 -> Bus Creator/1  "<PaO2>"
  rs_tehrani/1(Output) -> rs integrator/1(In1)
  Bus Selector1/1 -> Predicted Body Weight/1(height)  "<height>"
  Constant7/1 -> Bus Creator/6  "CvT;CO2;0"
  Constant/1 -> Divide/2
  Bus Selector/1 -> Lung volume model/1(Input1)  "<f>"
  FRC [L]/1 -> Lung volume model/2(Input2)  "FRC"
  Lung volume model/1(dv1) -> rs_tehrani/4(v)  "v"
  Constant1/1 -> Lung volume model/4(Input4)  "VD"
  Bus Selector2/1 -> Body surface estimate/1(height)  "<height>"
  Subtract/1 -> Divide/1
  Lung volume model/2(dv) -> rs_tehrani/5(dv+)  "dv+"
  QT12/1 -> rs_tehrani/6(Pamb*)  "Pamb"
  Constant5/1 -> Bus Creator/4  "CvB;CO2;0"
  Predicted Body Weight/1(Weight) -> Deadspace by PBW/1(Weight)  "PBW"
  Bus Selector8/1 -> Lung volume model/5(Input5)  "<lambda>"
  Constant4/1 -> Bus Creator/3  "CvB;O2;0"
  Body surface estimate/1(surface) -> cvs_bkst/4(body surface)  "surface"
  Bus Selector3/1 -> Display4/1, Bus Creator1/10, Initial contractility/1(H0)  "<H>"
  Initial contractility/2(SR;0) -> Initial RV contractility/1, Bus Creator1/6  "SR;0"
  Bus Selector2/2 -> Body surface estimate/2(Weight)  "<weight>"
  Input/1 -> Bus Selector11/1, Bus Selector10/1, Bus Selector8/1  "patientParams"
  Tissue-Brain fork ratio/1(QT/Qco) -> rs_tehrani/12(QT;0/Qco;0)
  Bus Creator/1 -> rs integrator/2(In2), rs_tehrani/2(Qco2)  "xrs;0"
  Bus Selector8/3 -> Composite shunt ratio/2(rho_2)  "<rho_int>"
  Input4/1 -> Bus Selector1/1, Bus Selector/1  "patientInput"
  Constant6/1 -> Bus Creator/5  "CvT;O2;0"
  Composite shunt ratio/1(rho) -> rs_tehrani/9(rho)  "rho"
  Bus Selector8/2 -> Composite shunt ratio/1(rho_1)  "<rho_ext>"
  Bus Selector6/1 -> rs_tehrani/7(Fi;O2)  "<FiO2>"
  Inspired CO2 fraction/1 -> rs_tehrani/8(Fi;CO2)  "Fi;CO2"
  Selector3/1 -> Total metabolic rate/1(MRT;O2)
  Selector4/1 -> Total metabolic rate/2(MRB;O2)
  Metabolic Parameters/1(Output) -> Selector3/1, rs_tehrani/10(QT8)
  Metabolic Parameters/2(Output1) -> Selector4/1, rs_tehrani/11(QT4)

== system ards_model/Predicted Body Weight/IfThenElse ==
  if : Inport  OutDataTypeStr=boolean
  then : Inport  Port=2
  else : Inport  Port=3
  Merge : Merge
  NOT : Logic  Operator=NOT  IconShape=distinctive  AllPortsSameDT=off  OutDataTypeStr=boolean
  Subsystem1 : Subsystem
  Subsystem2 : Subsystem
  out : Outport
  wires:
  then/1 -> Subsystem1/1(in)
  Subsystem2/1(out) -> Merge/2
  if/1 -> NOT/1, Subsystem1/Enable
  else/1 -> Subsystem2/1(in)
  Subsystem1/1(out) -> Merge/1
  NOT/1 -> Subsystem2/Enable
  Merge/1 -> out/1

== system ards_model/Ventilation Parameter completion/Pinsp by PEEP, VT, cRS ==
  PEEP : Inport  Unit=mbar
  VT : Inport  Port=2  Unit=L
  cRS : Inport  Port=3  Unit=mL/mbar
  Enable : EnablePort
  Add : Sum
  Divide1 : Product  Inputs=*/
  Gain : Gain  Gain=0.001
  Pinsp : Outport  Unit=mbar
  wires:
  Divide1/1 -> Add/2
  cRS/1 -> Gain/1
  PEEP/1 -> Add/1
  Add/1 -> Pinsp/1  "Pinsp"
  VT/1 -> Divide1/1
  Gain/1 -> Divide1/2

== system ards_model/Ventilation Parameter completion/Subsystem1 ==
  in : Inport
  Enable : EnablePort
  out : Outport
  wires:
  in/1 -> out/1

== system ards_model/Ventilation Parameter completion/Subsystem2 ==
  in : Inport
  Enable : EnablePort
  out : Outport
  wires:
  in/1 -> out/1

== system ards_model/Ventilation Parameter completion/Subsystem3 ==
  in : Inport
  Enable : EnablePort
  out : Outport
  wires:
  in/1 -> out/1

== system ards_model/Ventilation Parameter completion/Subsystem4 ==
  in : Inport
  Enable : EnablePort
  out : Outport
  wires:
  in/1 -> out/1

== system ards_model/Ventilation Parameter completion/Subsystem5 ==
  in : Inport
  Enable : EnablePort
  out : Outport
  wires:
  in/1 -> out/1

== system ards_model/Ventilation Parameter completion/VT by PEEP, Pinsp, cRS ==
  PEEP : Inport  Unit=mbar
  Pinsp : Inport  Port=2  Unit=mbar
  cRS : Inport  Port=3  Unit=mL/mbar
  Enable : EnablePort
  Gain : Gain  Gain=0.001
  Product : Product
  Subtract : Sum  Inputs=-+
  VT : Outport  Unit=L
  wires:
  Product/1 -> VT/1  "VT"
  Subtract/1 -> Product/1
  Pinsp/1 -> Subtract/2
  PEEP/1 -> Subtract/1
  cRS/1 -> Gain/1
  Gain/1 -> Product/2

== system ards_model/Ventilation Parameter completion/cRS by PEEP, Pinsp, VT ==
  PEEP : Inport  Unit=mbar
  Pinsp : Inport  Port=2  Unit=mbar
  VT : Inport  Port=3  Unit=L
  Enable : EnablePort
  Divide : Product  Inputs=*/
  Gain : Gain  Gain=1000
  Subtract1 : Sum  Inputs=+-
  cRS : Outport  Unit=mL/mbar
  wires:
  VT/1 -> Divide/1
  Subtract1/1 -> Divide/2
  Pinsp/1 -> Subtract1/1
  PEEP/1 -> Subtract1/2
  Divide/1 -> Gain/1  "cRS"
  Gain/1 -> cRS/1

== system ards_model/ards_classification/ARDS level score calculation ==
  severe : Inport
  moderate : Inport  Port=2
  mild : Inport  Port=3
  no : Inport  Port=4
  ARDS level score: mild ARDS : EditField  LabelPosition=Hide  ShowInitialText=on  Alignment=Center
  ARDS level score: moderate ARDS : EditField  LabelPosition=Hide  ShowInitialText=on  Alignment=Center
  ARDS level score: no ARDS : EditField  LabelPosition=Hide  ShowInitialText=on  Alignment=Center
  ARDS level score: severe ARDS : EditField  LabelPosition=Hide  ShowInitialText=on  Alignment=Center
  ARDS score: alpha : EditField  LabelPosition=Hide  ShowInitialText=on  Alignment=Center
  Add : Sum
  Constant : Constant
  Constant1 : Constant
  Constant2 : Constant  Value=0.9
  Constant3 : Constant  Value=0.7
  Constant4 : Constant  Value=0
  Gain : Gain  Gain=2
  Merge : Merge  Inputs=4
  Product : Product
  Subsystem : Subsystem
  Subsystem1 : Subsystem
  Subsystem2 : Subsystem
  Subsystem3 : Subsystem
  Subtract : Sum  Inputs=+-
  alpha : Constant  Value=0.05
  ards_level_score : Outport  Unit=1
  wires:
  severe/1 -> Subsystem/Enable
  Subsystem/1(out) -> Merge/1
  Constant3/1 -> Subsystem2/1(in)
  Subsystem3/1(out) -> Merge/4
  Subsystem2/1(out) -> Merge/3
  Subsystem1/1(out) -> Merge/2
  Constant1/1 -> Subtract/1
  mild/1 -> Subsystem2/Enable
  alpha/1 -> Gain/1, Add/1
  Constant2/1 -> Subsystem1/1(in)
  no/1 -> Subsystem3/Enable
  moderate/1 -> Subsystem1/Enable
  Add/1 -> ards_level_score/1  "ARDS_level_score"
  Constant/1 -> Subsystem/1(in)
  Constant4/1 -> Subsystem3/1(in)
  Merge/1 -> Product/2
  Product/1 -> Add/2
  Subtract/1 -> Product/1
  Gain/1 -> Subtract/2

== system ards_model/ards_classification/ARDS score calculation ==
  ARDS_level_score : Inport  Unit=1
  HF_score : Inport  Port=2  Unit=1
  ARDS score: HF score gain : EditField  LabelPosition=Hide  ShowInitialText=on  Alignment=Center
  Constant : Constant
  Gain : Gain  Gain=0.75
  Product : Product
  Subtract : Sum  Inputs=+-
  ARDS_score : Outport  Unit=1
  wires:
  HF_score/1 -> Gain/1
  Constant/1 -> Subtract/1
  Subtract/1 -> Product/2  "no_HF_score"
  ARDS_level_score/1 -> Product/1
  Gain/1 -> Subtract/2
  Product/1 -> ARDS_score/1  "ARDS_score"

== system ards_model/ards_classification/BNP_score ==
  note: BNP Score
      | depending on the BNP input value, this subsystem calculates a score between 0 and 1.
      | 0 means no heart failure, 1 means heart failure.
      | The parameter lambda sets a minimum error, limiting the result to the interval [lambda, 1-lambda].
      | BNP values below the rule-out bound (35 pg/mL) yield a minimum score (lambda).
      | BNP values above the rule-in bound (400 pg/mL) yield a maximum score (1-lambda).
      | For values inbetween, a linear slope is generated, determined by the above boundary values.
      |
      | Source for rule-out / rule-in bounds: Zwei kardiale Marker werden "erwachsen"
  BNP : Inport  Unit=pg/mL
  BNP rule-in bound [pg/mL] : Constant  Value=400
  BNP rule-out bound [pg/mL] : Constant  Value=35
  BNP score: alpha : Constant  Value=0.05
  Constant : Constant
  Subsystem2 : Subsystem  ReferencedSubsystem=linear_slope_score
  Subtract : Sum  Inputs=+-
  BNPscore : Outport  Unit=1
  wires:
  BNP rule-out bound [pg/mL]/1 -> Subsystem2/2  "bound_ruleOut"
  Subtract/1 -> Subsystem2/5  "beta"
  BNP/1 -> Subsystem2/1
  BNP rule-in bound [pg/mL]/1 -> Subsystem2/3  "bound_ruleIn"
  Constant/1 -> Subtract/1
  Subsystem2/1 -> BNPscore/1
  BNP score: alpha/1 -> Subsystem2/4, Subtract/2  "alpha"

== system ards_model/ards_classification/Berlin definition ==
  PEEP : Inport  Unit=mbar
  horowitz : Inport  Port=2  Unit=mmHg
  Input : Inport  Port=3  Unit=1
  Input1 : Inport  Port=4  Unit=m
  Pamb : Inport  Port=5  Unit=mmHg
  Display : Display
  NOT : Logic  Operator=NOT  IconShape=distinctive  AllPortsSameDT=off  OutDataTypeStr=boolean
  PEEP bound : Subsystem
  ards_level : Subsystem
  out_string : Outport
  nopeep : Outport  Port=2
  Out3 : Outport  Port=3
  Out4 : Outport  Port=4
  Out5 : Outport  Port=5
  Out6 : Outport  Port=6
  Out1 : Outport  Port=7
  wires:
  Pamb/1 -> ards_level/4(Pamb)  "Pamb"
  ards_level/3(no) -> Out6/1  "no"
  NOT/1 -> nopeep/1  "nopeep"
  horowitz/1 -> ards_level/1(horowitz)  "horowitz"
  PEEP/1 -> PEEP bound/1(PEEP)  "PEEP"
  ards_level/4(mild) -> Out5/1  "mild"
  ards_level/5(moderate) -> Out4/1  "moderate"
  PEEP bound/1(Out1) -> ards_level/5(Input), Display/1, NOT/1  "ispeep"
  ards_level/6(severe) -> Out3/1  "severe"
  ards_level/1(Out1) -> out_string/1  "ARDS_level"
  ards_level/2(ards) -> Out1/1  "ards"
  Input/1 -> ards_level/2(Fi;O2)  "Fi;O2"
  Input1/1 -> ards_level/3(altitude)  "altitude"

== system ards_model/ards_classification/HeartFrequency_score ==
  <H> : Inport
  Constant : Constant  Value=75
  Constant1 : Constant  Value=200
  Constant2 : Constant  Value=0.2
  Constant3 : Constant  Value=0.5
  Subsystem2 : Subsystem  ReferencedSubsystem=linear_slope_score
  H_score : Outport
  wires:
  Subsystem2/1 -> H_score/1  "H_score"
  Constant1/1 -> Subsystem2/3
  Constant3/1 -> Subsystem2/5
  Constant/1 -> Subsystem2/2
  Constant2/1 -> Subsystem2/4
  <H>/1 -> Subsystem2/1  "H"

== system ards_model/ards_classification/LVEF_score ==
  EFL : Inport  Unit=1
  Constant1 : Constant  Value=0.5
  Constant2 : Constant  Value=0.3
  Constant7 : Constant  Value=0.4
  Constant8 : Constant  Value=0.5
  Enabled Subsystem : Subsystem  TreatAsAtomicUnit=on
  Enabled Subsystem1 : Subsystem  TreatAsAtomicUnit=on
  Enabled Subsystem2 : Subsystem  TreatAsAtomicUnit=on
  GreaterThan : RelationalOperator  Operator=>  OutDataTypeStr=boolean  RndMeth=Simplest
  LVEF score: max score (at EF < 30%) : Constant  Value=0.95
  LVEF score: min score (at EF > 50%) : Constant  Value=0.05
  Less Than : RelationalOperator  Operator=<  OutDataTypeStr=boolean  RndMeth=Simplest
  Merge : Merge  Inputs=3
  NOR : Logic  Operator=NOR  IconShape=distinctive  AllPortsSameDT=off  OutDataTypeStr=boolean
  String Constant : StringConstant  String="\"reduced LVEF\""
  String Constant1 : StringConstant  String="\"moderate LVEF\""
  String Constant2 : StringConstant  String="\"preserved LVEF\""
  Subsystem2 : Subsystem  ReferencedSubsystem=linear_slope_score
  LVEF_score : Outport  Unit=1
  LVEF_level_string : Outport  Port=2  Unit=1
  wires:
  LVEF score: max score (at EF < 30%)/1 -> Subsystem2/4  "alpha"
  Subsystem2/1 -> LVEF_score/1
  EFL/1 -> Subsystem2/1, GreaterThan/1, Less Than/1
  Enabled Subsystem/1(Out1) -> Merge/1
  Enabled Subsystem1/1(Out1) -> Merge/2
  Enabled Subsystem2/1(Out1) -> Merge/3
  Merge/1 -> LVEF_level_string/1
  GreaterThan/1 -> Enabled Subsystem2/Enable, NOR/2
  Constant8/1 -> GreaterThan/2
  Constant7/1 -> Less Than/2
  Less Than/1 -> NOR/1, Enabled Subsystem/Enable
  String Constant/1 -> Enabled Subsystem/1(In1)
  String Constant2/1 -> Enabled Subsystem2/1(In1)
  String Constant1/1 -> Enabled Subsystem1/1(In1)
  NOR/1 -> Enabled Subsystem1/Enable
  Constant1/1 -> Subsystem2/3
  Constant2/1 -> Subsystem2/2
  LVEF score: min score (at EF > 50%)/1 -> Subsystem2/5  "beta"

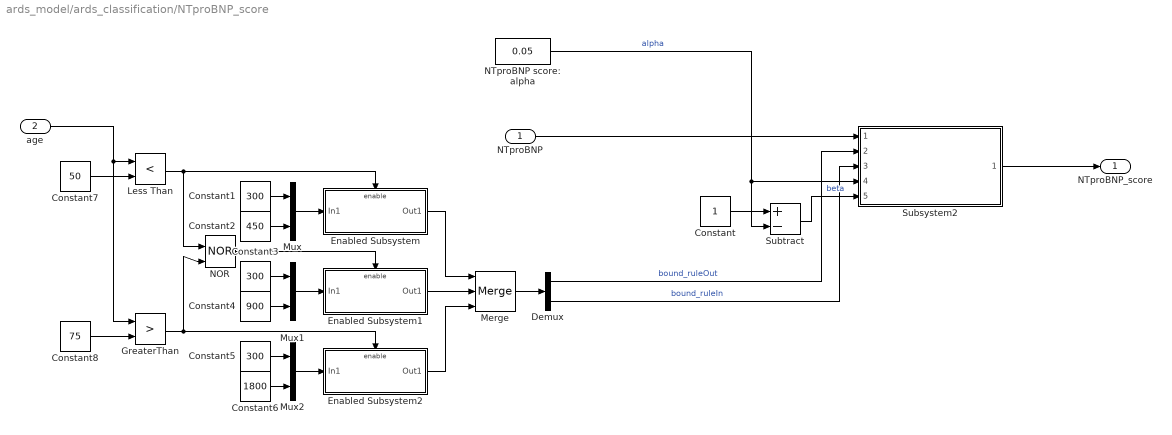
== system ards_model/ards_classification/NTproBNP_score ==
  NTproBNP : Inport  Unit=pg/mL
  age : Inport  Port=2
  Constant : Constant
  Constant1 : Constant  Value=300
  Constant2 : Constant  Value=450
  Constant3 : Constant  Value=300
  Constant4 : Constant  Value=900
  Constant5 : Constant  Value=300
  Constant6 : Constant  Value=1800
  Constant7 : Constant  Value=50
  Constant8 : Constant  Value=75
  Demux : Demux  Outputs=2
  Enabled Subsystem : Subsystem  TreatAsAtomicUnit=on
  Enabled Subsystem1 : Subsystem  TreatAsAtomicUnit=on
  Enabled Subsystem2 : Subsystem  TreatAsAtomicUnit=on
  GreaterThan : RelationalOperator  Operator=>  OutDataTypeStr=boolean  RndMeth=Simplest
  Less Than : RelationalOperator  Operator=<  OutDataTypeStr=boolean  RndMeth=Simplest
  Merge : Merge  Inputs=3
  Mux : Mux  Inputs=2
  Mux1 : Mux  Inputs=2
  Mux2 : Mux  Inputs=2
  NOR : Logic  Operator=NOR  IconShape=distinctive  AllPortsSameDT=off  OutDataTypeStr=boolean
  NTproBNP score: alpha : Constant  Value=0.05
  Subsystem2 : Subsystem  ReferencedSubsystem=linear_slope_score
  Subtract : Sum  Inputs=+-
  NTproBNP_score : Outport  Unit=1
  wires:
  NTproBNP score: alpha/1 -> Subtract/2, Subsystem2/4  "alpha"
  Subsystem2/1 -> NTproBNP_score/1
  Constant/1 -> Subtract/1
  Demux/2 -> Subsystem2/3  "bound_ruleIn"
  NTproBNP/1 -> Subsystem2/1
  Subtract/1 -> Subsystem2/5  "beta"
  Demux/1 -> Subsystem2/2  "bound_ruleOut"
  age/1 -> GreaterThan/1, Less Than/1
  Constant1/1 -> Mux/1
  Constant2/1 -> Mux/2
  Mux/1 -> Enabled Subsystem/1(In1)
  Enabled Subsystem/1(Out1) -> Merge/1
  Mux1/1 -> Enabled Subsystem1/1(In1)
  Constant4/1 -> Mux1/2
  Enabled Subsystem1/1(Out1) -> Merge/2
  Constant6/1 -> Mux2/2
  Mux2/1 -> Enabled Subsystem2/1(In1)
  Enabled Subsystem2/1(Out1) -> Merge/3
  Merge/1 -> Demux/1
  GreaterThan/1 -> NOR/2, Enabled Subsystem2/Enable
  Constant8/1 -> GreaterThan/2
  Constant7/1 -> Less Than/2
  Less Than/1 -> NOR/1, Enabled Subsystem/Enable
  NOR/1 -> Enabled Subsystem1/Enable
  Constant3/1 -> Mux1/1
  Constant5/1 -> Mux2/1

== system ards_model/ards_classification/Phf_score ==
  LVEF_score : Inport
  <H> : Inport  Port=2
  NTproBNP_score : Inport  Port=3
  Add : Sum  Inputs=+++
  Constant : Constant  Value=3
  Divide : Product  Inputs=*/
  Phf_score : Outport
  wires:
  Divide/1 -> Phf_score/1  "Phf_score"
  <H>/1 -> Add/1  "H"
  LVEF_score/1 -> Add/2
  NTproBNP_score/1 -> Add/3
  Add/1 -> Divide/1
  Constant/1 -> Divide/2

== system ards_model/ards_classification/RHF_risk_level ==
  RHF_score : Inport
  AND : Logic  IconShape=distinctive  AllPortsSameDT=off  OutDataTypeStr=boolean
  AND1 : Logic  IconShape=distinctive  AllPortsSameDT=off  OutDataTypeStr=boolean
  LessThan1 : RelationalOperator  Operator=<=  OutDataTypeStr=boolean  RndMeth=Simplest
  LessThan2 : RelationalOperator  Operator=<=  OutDataTypeStr=boolean  RndMeth=Simplest
  LessThan3 : RelationalOperator  Operator=<=  OutDataTypeStr=boolean  RndMeth=Simplest
  NOT : Logic  Operator=NOT  IconShape=distinctive  AllPortsSameDT=off  OutDataTypeStr=boolean
  NOT1 : Logic  Operator=NOT  IconShape=distinctive  AllPortsSameDT=off  OutDataTypeStr=boolean
  NOT2 : Logic  Operator=NOT  IconShape=distinctive  AllPortsSameDT=off  OutDataTypeStr=boolean
  high : Constant  Value=5
  low : Constant  Value=50
  moderate : Constant  Value=10
  ishigh : Outport
  ismoderate : Outport  Port=2
  islow : Outport  Port=3
  isminimal : Outport  Port=4
  wires:
  LessThan2/1 -> AND1/2, NOT2/1
  low/1 -> LessThan2/2
  RHF_score/1 -> LessThan2/1, LessThan3/1, LessThan1/1
  LessThan3/1 -> AND/2, NOT1/1
  NOT/1 -> AND/1
  moderate/1 -> LessThan3/2
  high/1 -> LessThan1/2
  NOT1/1 -> AND1/1
  LessThan1/1 -> ishigh/1, NOT/1  "high"
  NOT2/1 -> isminimal/1  "minimal"
  AND1/1 -> islow/1  "low"
  AND/1 -> ismoderate/1  "moderate"

== system ards_model/ards_classification/RHF_risk_level_string ==
  In1 : Inport
  In2 : Inport  Port=2
  In3 : Inport  Port=3
  In4 : Inport  Port=4
  Merge : Merge  Inputs=4
  String Constant : StringConstant  String="\"high\""
  String Constant1 : StringConstant  String="\"moderate\""
  String Constant2 : StringConstant  String="\"low\""
  String Constant3 : StringConstant  String="\"minimal\""
  Subsystem : Subsystem
  Subsystem1 : Subsystem
  Subsystem2 : Subsystem
  Subsystem3 : Subsystem
  ards_level : Outport
  wires:
  Subsystem1/1(out) -> Merge/2
  Merge/1 -> ards_level/1  "RHFscore_level"
  Subsystem/1(out) -> Merge/1
  In1/1 -> Subsystem/Enable  "high"
  Subsystem3/1(out) -> Merge/4
  Subsystem2/1(out) -> Merge/3
  String Constant/1 -> Subsystem/1(in)
  String Constant1/1 -> Subsystem1/1(in)
  In2/1 -> Subsystem1/Enable  "moderate"
  In3/1 -> Subsystem2/Enable  "low"
  In4/1 -> Subsystem3/Enable  "minimal"
  String Constant2/1 -> Subsystem2/1(in)
  String Constant3/1 -> Subsystem3/1(in)

== system ards_model/ards_classification/RHF_score ==
  EFL : Inport  OutDataTypeStr=double  Unit=1
  BNP2 : Inport  Port=2  Unit=g/dL
  BNP1 : Inport  Port=3  Unit=pg/mL
  eGFR : Inport  Port=4
  Gain : Gain  Gain=100
  Product : Product  Inputs=***/
  RHFscore : Outport
  wires:
  Gain/1 -> Product/1  "EFL [%]"
  Product/1 -> RHFscore/1  "RHF_score"
  EFL/1 -> Gain/1
  BNP2/1 -> Product/2  "Hb"
  BNP1/1 -> Product/4  "NTproBNP"
  eGFR/1 -> Product/3

== system ards_model/ards_classification/eGFR_CKD-EPI ==
  note: CKD-EPI Equation for eGFR
      | (estimated Glomerular Filtration Rate)
      |
      | GFR = 141 × min (Scr /κ, 1)^α × max(Scr /κ, 1)^(-1.209) × 0.993^age × 1.018 [if female] × 1.159 [if black]
      | where:
      | Scr is serum creatinine in mg/dL,
      | κ is 0.7 for females and 0.9 for males,
      | α is -0.329 for females and -0.411 for males,
      |
      | Source
  Scr : Inport  Unit=mg/dL
  age : Inport  Port=2
  female : Inport  Port=3
  black : Inport  Port=4
  Constant : Constant  Value=141
  Constant2 : Constant
  Constant3 : Constant  Value=-1.209
  Constant4 : Constant  Value=0.993
  Divide : Product  Inputs=*/
  Min : MinMax  Inputs=2
  Min1 : MinMax  Function=max  Inputs=2
  Power : Math  Operator=pow  SaturateOnIntegerOverflow=on
  Power1 : Math  Operator=pow  SaturateOnIntegerOverflow=on
  Power2 : Math  Operator=pow  SaturateOnIntegerOverflow=on
  Product1 : Product  Inputs=6
  alpha : Subsystem
  kappa : Subsystem
  sex factor : Subsystem
  skin color factor : Subsystem
  eGFR : Outport  Unit=mL/min
  wires:
  Constant2/1 -> Min1/2, Min/1
  kappa/1(Out1) -> Divide/2  "kappa"
  Min1/1 -> Power1/1
  female/1 -> kappa/1(In1), alpha/1(In1), sex factor/1(In1)
  Power/1 -> Product1/2
  Scr/1 -> Divide/1
  Product1/1 -> eGFR/1  "eGFR"
  Min/1 -> Power/1
  Divide/1 -> Min1/1, Min/2
  Constant3/1 -> Power1/2
  alpha/1(Out1) -> Power/2  "alpha"
  skin color factor/1(Out1) -> Product1/6
  black/1 -> skin color factor/1(In1)
  Power1/1 -> Product1/3
  Power2/1 -> Product1/4
  Constant/1 -> Product1/1
  sex factor/1(Out1) -> Product1/5
  Constant4/1 -> Power2/1
  age/1 -> Power2/2

== system ards_model/ards_classification/logFon_score ==
  note: 0.0212 * BUN − 0.0192 * SBP + 0.0131 * H + 0.0288 * age − 4.72
      | ["Risk Stratification for In-Hospital Mortality in Acutely Decompensated Heart Failure"]
  patientState : Inport
  patientInput : Inport  Port=2
  Add : Sum  Inputs=5
  Bus Selector10 : BusSelector  OutputSignals=cvs.H
  Bus Selector11 : BusSelector  OutputSignals=height,weight
  Bus Selector8 : BusSelector  OutputSignals=cvs.Pas,cvs.H,cvs.LV.Vstr
  Bus Selector9 : BusSelector  OutputSignals=BUN,age
  Compliance : Subsystem
  Constant : Constant  Value=-4.72
  Constant1 : Constant  Value=100
  Display1 : Display
  Display6 : Display
  Gain : Gain  Gain=0.0212
  Gain1 : Gain  Gain=-0.0192
  Gain2 : Gain  Gain=0.0131
  Gain3 : Gain  Gain=0.0288
  Power of 10 : Math  Operator=10^u  SaturateOnIntegerOverflow=on
  Product : Product
  To Workspace1 : ToWorkspace  VariableName=Psystas  SaveFormat=Timeseries  SampleTime=-1
  To Workspace2 : ToWorkspace  VariableName=Pdiastas  SaveFormat=Timeseries  SampleTime=-1
  peak Pas : Subsystem
  pFon : Outport
  wires:
  Bus Selector9/1 -> Gain/1  "<BUN>"
  patientInput/1 -> Bus Selector9/1, Bus Selector11/1
  Bus Selector11/1 -> Compliance/1(<height>)  "<height>"
  Gain1/1 -> Add/2
  Gain2/1 -> Add/3
  Bus Selector8/1 -> peak Pas/1(<Pas>)  "<Pas>"
  Bus Selector11/2 -> Compliance/2(<weight>)  "<weight>"
  Bus Selector8/2 -> peak Pas/2(<H>)  "<H>"
  Add/1 -> Display6/1, Power of 10/1  "logFon_score"
  Constant/1 -> Add/5
  patientState/1 -> Bus Selector10/1, Bus Selector8/1
  Bus Selector8/3 -> peak Pas/3(<Vstr>)  "<Vstr>"
  Compliance/1(cas) -> peak Pas/4(cas)  "cas"
  Gain/1 -> Add/1
  Bus Selector10/1 -> Gain2/1  "<H>"
  peak Pas/2(Pas;syst) -> Gain1/1, To Workspace1/1  "Pas;syst"
  Bus Selector9/2 -> Gain3/1  "<age>"
  Gain3/1 -> Add/4
  peak Pas/1(Pas;diast) -> To Workspace2/1
  Power of 10/1 -> Product/1, Display1/1
  Product/1 -> pFon/1
  Constant1/1 -> Product/2

== system ards_model/main-model/Body surface estimate ==
  note: s = 0.007184 w^0.425 h^0.725
      |
      | source: CVRS ch 1.6.1 [Du Bois’ formula (Keidl, 1985, p. 377)]
      | WolframAlpha
  height : Inport  Unit=m
  Weight : Inport  Port=2  Unit=kg
  Constant1 : Constant  Value=0.007184
  Constant2 : Constant  Value=0.725
  Constant3 : Constant  Value=0.425
  Gain : Gain  Gain=100
  Power : Math  Operator=pow  SaturateOnIntegerOverflow=on
  Power1 : Math  Operator=pow  SaturateOnIntegerOverflow=on
  Product2 : Product  Inputs=***
  surface : Outport  Unit=m^2
  wires:
  Power1/1 -> Product2/2
  Constant2/1 -> Power/2
  Constant1/1 -> Product2/3
  Product2/1 -> surface/1  "surface"
  Constant3/1 -> Power1/2
  Power/1 -> Product2/1
  Weight/1 -> Power1/1  "weight"
  height/1 -> Gain/1  "height"
  Gain/1 -> Power/1  "height [cm]"

== system ards_model/main-model/Composite shunt ratio ==
  rho_1 : Inport
  rho_2 : Inport  Port=2
  Add1 : Sum
  Constant : Constant
  Product : Product
  Subtract : Sum  Inputs=+-
  rho : Outport
  wires:
  rho_1/1 -> Add1/1, Subtract/2
  Product/1 -> Add1/2
  Add1/1 -> rho/1  "rho"
  Subtract/1 -> Product/2
  rho_2/1 -> Product/1
  Constant/1 -> Subtract/1
